simulink model "ee_solenoid_fem"  (R2022a)
settings: Solver=VariableStepAuto  StartTime=0.0  StopTime=0.1  FixedStep=2e-5  MaxStep=0.001  RelTol=1e-3  EnableMultiTasking=on
PreLoadFcn:
  | load ee_solenoid_fem_data
StopFcn:
  | ee_addSimlogTimeStamp(bdroot)
values from neighbouring files (symbols this model uses):
  lambda = 20    [ee_solenoid_fem_params.m]
  mass = 0.1    [ee_solenoid_fem_params.m]
  R = 14    [ee_solenoid_fem_params.m]
libraries: fl_lib x27, fl_ps_legacy_lib x10, nesl_utility x7, ee_lib x1
CloseFcn:
  | try,close(h1_ee_solenoid_fem),end
  | clear h1_ee_solenoid_fem
  | try,close(h2_ee_solenoid_fem),end
  | clear h2_ee_solenoid_fem
  | try,close(h3_ee_solenoid_fem),end
  | clear h3_ee_solenoid_fem
  | try,close(h4_ee_solenoid_fem),end
  | clear h4_ee_solenoid_fem
  | try,close(h5_ee_solenoid_fem),end
  | clear h5_ee_solenoid_fem
  | 
  | clear simlog_ee_solenoid_fem
  | clear logsout_ee_solenoid_fem
  | clear Coeff L R X a b current dLdx data_coeff dflux_dx dflux_dx1 dflux_dx2 dfluxdi dfluxdx f_c flux_linkage flux_linkage2 flux_x force force2 force_x i lambda mass oo ord p tout x x0 xmax xmin zz
Description:
  | Solenoid Parameterized with FEM Data
settings Model: Creator=The MathWorks, Inc.  LastModifiedBy=whatastarrynight
settings SolverCC: AlgebraicLoopSolver=TrustRegion
settings DataIOCC: LimitDataPoints=on  MaxDataPoints=10000  SaveFormat=Array  ReturnWorkspaceOutputs=off  SignalLoggingName=logsout_ee_solenoid_fem
settings OptimizationCC: ExpressionDepthLimit=2147483647  InitFltsAndDblsToZero=on  LifeSpan=inf
settings DebuggingCC: SaveWithParameterizedLinksMsg=none  UnderspecifiedInitializationDetection=Classic  MergeDetectMultiDrivingBlocksExec=none  SignalResolutionControl=TryResolveAllWithWarning  SolverPrmCheckMsg=warning  FcnCallInpInsideContextMsg=warning  UnconnectedInputMsg=warning  UnconnectedOutputMsg=warning  UnconnectedLineMsg=warning  StateNameClashWarn=warning  SFUnexpectedBacktrackingDiag=warning  SFNoUnconditionalDefaultTransitionDiag=warning  SFExecutionAtInitializationDiag=none  SFMachineParentedDataDiag=warning  ArithmeticOperatorsInVariantConditions=warning
settings HardwareCC: ProdBitPerPointer=32  ProdBitPerSizeT=32  ProdBitPerPtrDiffT=32  ProdLargestAtomicFloat=None  ProdIntDivRoundTo=Undefined  ProdEndianess=Unspecified  ProdWordSize=32  ProdHWDeviceType=32-bit Generic
settings ModelReferenceCC: PropagateSignalLabelsOutOfModel=off
settings SFSimCC: SimUseLocalCustomCode=off  CustomCodeUndefinedFunction=UseInterfaceOnly
settings RTWCC: RTWUseLocalCustomCode=off  DLArmComputeVersion=19.05
settings CodeAppCC: StateflowObjectComments=on
settings GRTTargetCC: TargetFcnLib=ansi_tfl_tmw.mat  TargetLangStandard=C89/C90 (ANSI)  CombineOutputUpdateFcns=off  GRTInterface=on
settings ConfigComp: CovMetricSettings=dw  CovSaveCumulativeToWorkspaceVar=on  CovSaveSingleToWorkspaceVar=on  CovExternalEMLEnable=off  CovSFcnEnable=off
settings SimscapeCC: SimscapeLogType=all  SimscapeLogSimulationStatistics=on  SimscapeLogToSDI=on  SimscapeLogName=simlog_ee_solenoid_fem  SimscapeLogDataHistory=10000

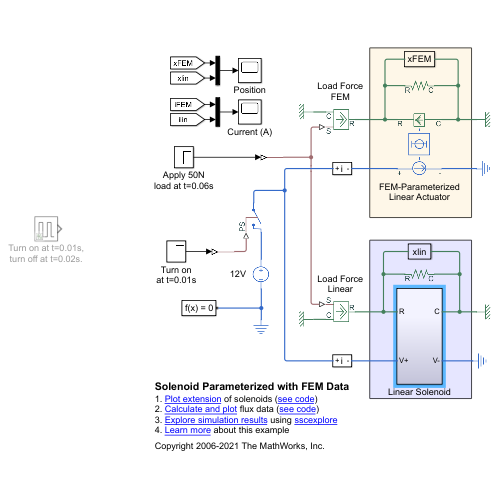
[thumbnail: Simulink's stored preview of the top-level diagram]
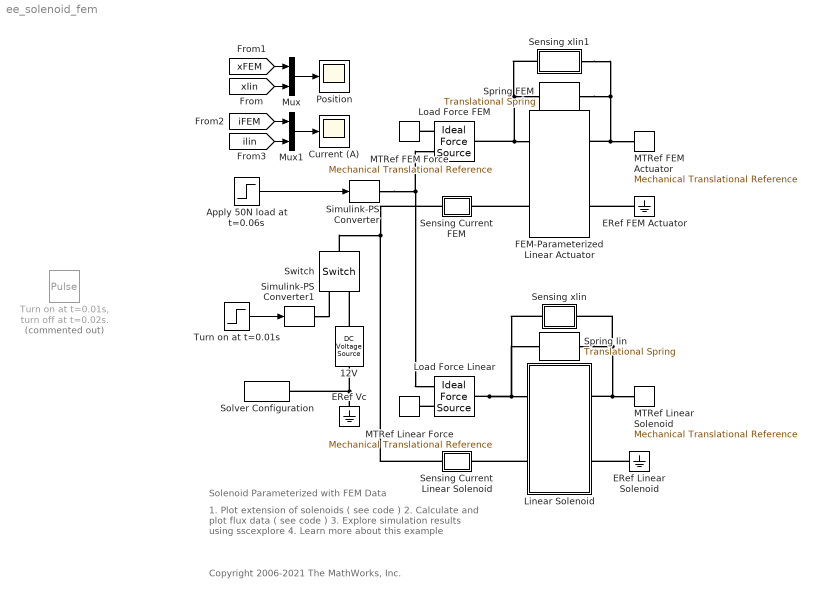
== system ee_solenoid_fem ==
  note: Solenoid Parameterized with FEM Data
  note: 1. Plot extension of solenoids ( see code )
      | 2. Calculate and plot flux data ( see code )
      | 3. Explore simulation results using sscexplore
      | 4. Learn more about this example
  note: Copyright 2006-2021 The MathWorks, Inc.
  12V : fl_lib/Electrical/Electrical Sources/DC Voltage Source  v0=12 V
      settings: SourceProductBaseCode=PW,SS,VE
  Apply 50N load at t=0.06s : Step  Time=0.06  After=50  SampleTime=0
  Current (A) : Scope
  ERef FEM Actuator : fl_lib/Electrical/Electrical Elements/Electrical Reference
      settings: SourceProductBaseCode=PW,SS,VE
  ERef Linear Solenoid : fl_lib/Electrical/Electrical Elements/Electrical Reference
      settings: SourceProductBaseCode=PW,SS,VE
  ERef Vc : fl_lib/Electrical/Electrical Elements/Electrical Reference
      settings: SourceProductBaseCode=PW,SS,VE
  FEM-Parameterized Linear Actuator : ee_lib/Electromechanical/Mechatronic Actuators/FEM-Parameterized Linear Actuator  src_type=2  iVec=current A  xVec=x m  dfluxdiMatrix=dfluxdi Wb/A  dfluxdxMatrix=dfluxdx Wb/m  FluxMatrix=flux_linkage Wb  calculate_force_matrix=ee.enum.enable.no  ForceMatrix=force N  cyclic=1  interp_method=1  extrap_method=1  R1=R Ohm  Rm=inf Ohm  lam=lambda N/(m/s)  Mass=mass kg  Xmin=xmin m  Xmax=xmax m  K_endstop=1e10 N/m  D_endstop=1e5 N/(m/s)  i_specify=off  i_priority=None  i=0 A  i_nominal_specify=off  i_nominal_unit=A  i_nominal_value=1  F_specify=off  F_priority=None  F=0 N  F_nominal_specify=off  F_nominal_unit=N  F_nominal_value=1  x_specify=on  x_priority=High  x=x0 m  x_nominal_specify=off  x_nominal_unit=mm  x_nominal_value=1  vel_specify=on  vel_priority=Low  vel=0 mm/s  vel_nominal_specify=off  vel_nominal_unit=mm/s  vel_nominal_value=1  magnetic_force_specify=off  magnetic_force_priority=None  magnetic_force=0 N  magnetic_force_nominal_specify=off  magnetic_force_nominal_unit=N  magnetic_force_nominal_value=1  alpha=3.93e-3 1/K  Tmeas=25 degC  thermal_mass=100 J/K  T_specify=off  T_priority=High  T=300 K  T_nominal_specify=off  T_nominal_unit=K  T_nominal_value=1
      settings: SourceProductBaseCode=PS  InternalSimscapePortConfiguration="{\"Bottom\":[],\"Left\":[{\"id\":\"p\",\"label\":\"+\",\"type\":\"foundation.electrical.electrical\"},{\"id\":\"R\",\"label\":\"R\",\"type\":\"foundation.mechanical.translational.translational\"}],\"Right\":[{\"id\":\"n\",\"label\":\"-\",\"type\":\"foundation.electrical.electrical\"},{\"id\":\"C\",\"label\":\"C\",\"type\":\"foundation.mechanical.translational.translational\"}],\"Top\":[]}"
  Linear Solenoid : Subsystem
  Load Force FEM : fl_lib/Mechanical/Mechanical Sources/Ideal Force Source
      settings: SourceProductBaseCode=PW,SS,VE
  Load Force Linear : fl_lib/Mechanical/Mechanical Sources/Ideal Force Source
      settings: SourceProductBaseCode=PW,SS,VE
  MTRef Linear Force : fl_lib/Mechanical/Translational Elements/Mechanical Translational Reference
      settings: SourceProductBaseCode=PW,SS,VE
  MTRef FEM Actuator : fl_lib/Mechanical/Translational Elements/Mechanical Translational Reference
      settings: SourceProductBaseCode=PW,SS,VE
  MTRef FEM Force : fl_lib/Mechanical/Translational Elements/Mechanical Translational Reference
      settings: SourceProductBaseCode=PW,SS,VE
  MTRef Linear Solenoid : fl_lib/Mechanical/Translational Elements/Mechanical Translational Reference
      settings: SourceProductBaseCode=PW,SS,VE
  Mux : Mux  Inputs=2
  Mux1 : Mux  Inputs=2
  Position : Scope
  Sensing Current FEM : Subsystem
      mask Display: disp('i')
  Sensing Current Linear Solenoid : Subsystem
      mask Display: disp('i')
  Sensing xlin : Subsystem
      mask Display: disp('xlin')
  Sensing xlin1 : Subsystem
      mask Display: disp('xFEM')
  Simulink-PS Converter : nesl_utility/Simulink-PS Converter  PhysicalDomain=network_engine_domain  SubClassName=ps_input  LeftPortType=input  RightPortType=output  PseudoPeriodic=off  Frequencies=[]  NoiseDistribution=none  NoiseParameters=[]  Unit=1  AffineConversion=off  FilteringAndDerivatives=zero  SimscapeFilterOrder=1  InputFilterTimeConstant=.001  UdotUserProvided=0
      settings: SourceProductBaseCode=SS,PW,VE
  Simulink-PS Converter1 : nesl_utility/Simulink-PS Converter  PhysicalDomain=network_engine_domain  SubClassName=ps_input  LeftPortType=input  RightPortType=output  PseudoPeriodic=off  Frequencies=[]  NoiseDistribution=none  NoiseParameters=[]  Unit=1  AffineConversion=off  FilteringAndDerivatives=zero  SimscapeFilterOrder=1  InputFilterTimeConstant=.001  UdotUserProvided=0
      settings: SourceProductBaseCode=SS,PW,VE
  Solver Configuration : nesl_utility/Solver Configuration  PhysicalDomain=network_engine_domain  SubClassName=solver  LeftPortType=input  RightPortType=generic  Tones=[]  Harmonics=[]  SimulateNoise=off  Profile=off  UseLocalSampling=off  EnableSwitchedLinearOptims=on  FrequencyDomain=off  UseCCode=off  RelTol=0.001  AbsTol=1e-06  MinStep=1e-09  ToWorkspace=off  RevertToSquareIcSolve=off  NumHomotopyIterations=100  PhasorMode=off  PhasorModeNumHarmonics=1  IndexReductionMethod=DerivativeReplacement  DoDC=off  ResidualTolerance=1e-9  UseLocalSolver=off  LocalSolverChoice=NE_TRAPEZOIDAL_ADVANCER  LocalSolverSampleTime=2e-5  DoFixedCost=off  MaxNonlinIter=12  MaxModeIter=2  ComputeImpulses=off  ImpulseIterations=2  LinearAlgebra=auto  LinearAlgebraNumThread=0  EquationFormulation=NE_TIME_EF  DelaysMemoryBudget=1024  AutomaticFiltering=on  FilteringTimeConstant=0.001  PartitionStorageMethod=AS_NEEDED  PartitionMemoryBudget=1024  PartitionMethod=FAST
      settings: SourceProductBaseCode=SS,PW,VE
  Spring FEM : fl_lib/Mechanical/Translational Elements/Translational Spring  spr_rate=200 N/m  v_specify=off  v_priority=High  v=0 m/s  v_nominal_specify=off  v_nominal_unit=m/s  v_nominal_value=1  f_specify=off  f_priority=High  f=0 N  f_nominal_specify=off  f_nominal_unit=N  f_nominal_value=1  x_specify=on  x_priority=High  x=0 mm  x_nominal_specify=off  x_nominal_unit=m  x_nominal_value=1
      settings: SourceProductBaseCode=PW,SS,VE
  Spring lin : fl_lib/Mechanical/Translational Elements/Translational Spring  spr_rate=200 N/m  v_specify=off  v_priority=High  v=0 m/s  v_nominal_specify=off  v_nominal_unit=m/s  v_nominal_value=1  f_specify=off  f_priority=High  f=0 N  f_nominal_specify=off  f_nominal_unit=N  f_nominal_value=1  x_specify=on  x_priority=High  x=0 mm  x_nominal_specify=off  x_nominal_unit=m  x_nominal_value=1
      settings: SourceProductBaseCode=PW,SS,VE
  Switch : fl_lib/Electrical/Electrical Elements/Switch  R_closed=0.01 Ohm  G_open=1e-8 1/Ohm  Threshold=0  i_specify=off  i_priority=High  i=0 A  i_nominal_specify=off  i_nominal_unit=A  i_nominal_value=1  v_specify=off  v_priority=High  v=0 V  v_nominal_specify=off  v_nominal_unit=V  v_nominal_value=1
      settings: SourceProductBaseCode=PW,SS,VE
  Turn on at t=0.01s : Step  Time=0.01  SampleTime=0
  "Turn on at t=0.01s, turn off at t=0.02s." : DiscretePulseGenerator  Commented=on  PulseType=Time based  Period=0.1  PulseWidth=10  PhaseDelay=0.01
  wires:
  Apply 50N load at t=0.06s/1 -> Simulink-PS Converter/1
  Mux/1 -> Position/1
  Mux1/1 -> Current (A)/1
  [xlin] -> Mux/2
  [xFEM] -> Mux/1
  [iFEM] -> Mux1/1
  [ilin] -> Mux1/2
  Turn on at t=0.01s/1 -> Simulink-PS Converter1/1
  connections:
  Linear Solenoid/LConn2 -- Sensing Current Linear Solenoid/RConn1
  Simulink-PS Converter1/RConn1 -- Switch/RConn1
  12V/LConn1 -- Switch/RConn2
  ERef Vc/LConn1 -- 12V/RConn1 -- Solver Configuration/RConn1
  ERef FEM Actuator/LConn1 -- FEM-Parameterized Linear Actuator/RConn1
  FEM-Parameterized Linear Actuator/LConn2 -- Load Force FEM/LConn1 -- Sensing xlin1/LConn1 -- Spring FEM/LConn1
  Spring FEM/RConn1 -- Sensing xlin1/RConn1 -- MTRef FEM Actuator/LConn1 -- FEM-Parameterized Linear Actuator/RConn2
  Load Force FEM/RConn2 -- MTRef FEM Force/LConn1
  Load Force Linear/RConn2 -- MTRef Linear Force/LConn1
  Simulink-PS Converter/RConn1 -- Load Force FEM/RConn1 -- Load Force Linear/RConn1
  Spring lin/RConn1 -- Sensing xlin/RConn1 -- MTRef Linear Solenoid/LConn1 -- Linear Solenoid/RConn1
  ERef Linear Solenoid/LConn1 -- Linear Solenoid/RConn2
  Load Force Linear/LConn1 -- Sensing xlin/LConn1 -- Spring lin/LConn1 -- Linear Solenoid/LConn1
  FEM-Parameterized Linear Actuator/LConn1 -- Sensing Current FEM/RConn1
  Sensing Current FEM/LConn1 -- Sensing Current Linear Solenoid/LConn1 -- Switch/LConn1

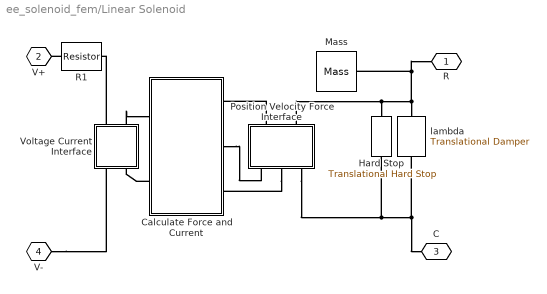
== system ee_solenoid_fem/Linear Solenoid ==
  Calculate Force and Current : Subsystem
  Hard Stop : fl_lib/Mechanical/Translational Elements/Translational Hard Stop  upper_bnd=xmax m  lower_bnd=xmin m  stiff_up=1e+10 N/m  stiff_low=1e+10 N/m  D_up=1e5 N/(m/s)  D_low=1e5 N/(m/s)  model=3  transition=0.1 mm  v_specify=off  v_priority=High  v=0 m/s  v_nominal_specify=off  v_nominal_unit=m/s  v_nominal_value=1  f_specify=off  f_priority=High  f=0 N  f_nominal_specify=off  f_nominal_unit=N  f_nominal_value=1  x_specify=on  x_priority=High  x=x0 m  x_nominal_specify=off  x_nominal_unit=m  x_nominal_value=1
      settings: SourceProductBaseCode=PW,SS,VE
  Mass : fl_lib/Mechanical/Translational Elements/Mass  mass=mass kg  num_ports=foundation.enum.numPorts2.one  v_specify=on  v_priority=High  v=0 m/s  v_nominal_specify=off  v_nominal_unit=m/s  v_nominal_value=1  f_specify=off  f_priority=High  f=0 N  f_nominal_specify=off  f_nominal_unit=N  f_nominal_value=1
      settings: SourceProductBaseCode=PW,SS,VE
  Position Velocity Force Interface : Subsystem
  R1 : fl_lib/Electrical/Electrical Elements/Resistor  R=R Ohm  i_specify=off  i_priority=High  i=0 A  i_nominal_specify=off  i_nominal_unit=A  i_nominal_value=1  v_specify=off  v_priority=High  v=0 V  v_nominal_specify=off  v_nominal_unit=V  v_nominal_value=1
      settings: SourceProductBaseCode=PW,SS,VE
  Voltage Current Interface : Subsystem
  lambda : fl_lib/Mechanical/Translational Elements/Translational Damper  D=lambda N/(m/s)  v_specify=off  v_priority=High  v=0 m/s  v_nominal_specify=off  v_nominal_unit=m/s  v_nominal_value=1  f_specify=off  f_priority=High  f=0 N  f_nominal_specify=off  f_nominal_unit=N  f_nominal_value=1
      settings: SourceProductBaseCode=PW,SS,VE
  R : PMIOPort  Side=Left
  V+ : PMIOPort  Port=2  Side=Left
  C : PMIOPort  Port=3  Side=Right
  V- : PMIOPort  Port=4  Side=Right
  connections:
  Hard Stop/RConn1 -- lambda/RConn1 -- C/RConn1 -- Position Velocity Force Interface/RConn3
  R1/LConn1 -- V+/RConn1
  lambda/LConn1 -- R/RConn1 -- Mass/LConn1 -- Position Velocity Force Interface/LConn2 -- Hard Stop/LConn1
  Position Velocity Force Interface/LConn1 -- Calculate Force and Current/RConn1
  Calculate Force and Current/RConn2 -- Position Velocity Force Interface/RConn1
  Position Velocity Force Interface/RConn2 -- Calculate Force and Current/RConn3
  Voltage Current Interface/LConn1 -- R1/RConn1
  V-/RConn1 -- Voltage Current Interface/RConn1
  Voltage Current Interface/LConn2 -- Calculate Force and Current/LConn1
  Calculate Force and Current/LConn2 -- Voltage Current Interface/RConn2

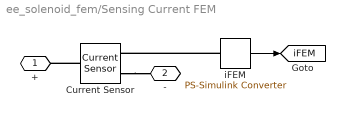
== system ee_solenoid_fem/Sensing Current FEM ==
  Current Sensor : fl_lib/Electrical/Electrical Sensors/Current Sensor
      settings: SourceProductBaseCode=PW,SS,VE
  iFEM : nesl_utility/PS-Simulink Converter  PhysicalDomain=network_engine_domain  SubClassName=ps_output  LeftPortType=input  RightPortType=output  PseudoPeriodic=off  Frequencies=[]  VectorFormat=1-D array  Unit=1  AffineConversion=off
      settings: SourceProductBaseCode=SS,PW,VE
  + : PMIOPort  Side=Left
  - : PMIOPort  Port=2  Side=Right
  tag scope: iFEM=global
  wires:
  iFEM/1 -> [iFEM]
  connections:
  iFEM/LConn1 -- Current Sensor/RConn1
  Current Sensor/LConn1 -- +/RConn1
  Current Sensor/RConn2 -- -/RConn1

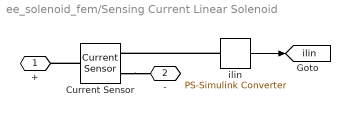
== system ee_solenoid_fem/Sensing Current Linear Solenoid ==
  Current Sensor : fl_lib/Electrical/Electrical Sensors/Current Sensor
      settings: SourceProductBaseCode=PW,SS,VE
  ilin : nesl_utility/PS-Simulink Converter  PhysicalDomain=network_engine_domain  SubClassName=ps_output  LeftPortType=input  RightPortType=output  PseudoPeriodic=off  Frequencies=[]  VectorFormat=1-D array  Unit=1  AffineConversion=off
      settings: SourceProductBaseCode=SS,PW,VE
  + : PMIOPort  Side=Left
  - : PMIOPort  Port=2  Side=Right
  tag scope: ilin=global
  wires:
  ilin/1 -> [ilin]
  connections:
  Current Sensor/RConn2 -- -/RConn1
  Current Sensor/LConn1 -- +/RConn1
  ilin/LConn1 -- Current Sensor/RConn1

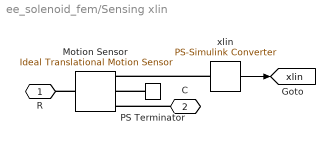
== system ee_solenoid_fem/Sensing xlin ==
  Motion Sensor : fl_lib/Mechanical/Mechanical Sensors/Ideal Translational Motion Sensor  offset=x0 m
      settings: SourceProductBaseCode=PW,SS,VE
  PS Terminator : fl_lib/Physical Signals/Sinks/PS Terminator
      settings: SourceProductBaseCode=PW,SS,VE
  xlin : nesl_utility/PS-Simulink Converter  PhysicalDomain=network_engine_domain  SubClassName=ps_output  LeftPortType=input  RightPortType=output  PseudoPeriodic=off  Frequencies=[]  VectorFormat=1-D array  Unit=mm  AffineConversion=off
      settings: SourceProductBaseCode=SS,PW,VE
  R : PMIOPort  Side=Left
  C : PMIOPort  Port=2  Side=Right
  tag scope: xlin=global
  wires:
  xlin/1 -> [xlin]
  connections:
  C/RConn1 -- Motion Sensor/RConn1
  PS Terminator/LConn1 -- Motion Sensor/RConn2
  Motion Sensor/LConn1 -- R/RConn1
  xlin/LConn1 -- Motion Sensor/RConn3

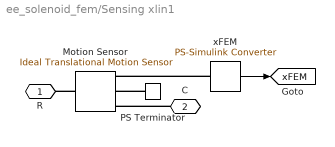
== system ee_solenoid_fem/Sensing xlin1 ==
  Motion Sensor : fl_lib/Mechanical/Mechanical Sensors/Ideal Translational Motion Sensor  offset=x0 m
      settings: SourceProductBaseCode=PW,SS,VE
  PS Terminator : fl_lib/Physical Signals/Sinks/PS Terminator
      settings: SourceProductBaseCode=PW,SS,VE
  xFEM : nesl_utility/PS-Simulink Converter  PhysicalDomain=network_engine_domain  SubClassName=ps_output  LeftPortType=input  RightPortType=output  PseudoPeriodic=off  Frequencies=[]  VectorFormat=1-D array  Unit=mm  AffineConversion=off
      settings: SourceProductBaseCode=SS,PW,VE
  R : PMIOPort  Side=Left
  C : PMIOPort  Port=2  Side=Right
  tag scope: xFEM=global
  wires:
  xFEM/1 -> [xFEM]
  connections:
  xFEM/LConn1 -- Motion Sensor/RConn3
  Motion Sensor/LConn1 -- R/RConn1
  PS Terminator/LConn1 -- Motion Sensor/RConn2
  C/RConn1 -- Motion Sensor/RConn1

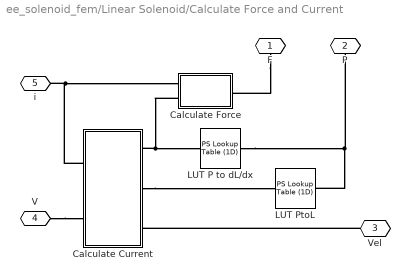
== system ee_solenoid_fem/Linear Solenoid/Calculate Force and Current ==
  Calculate Current : Subsystem
  Calculate Force : Subsystem
  LUT P to dL/dx : fl_ps_legacy_lib/Legacy Physical Signals/Lookup Tables/PS Lookup Table (1D)  x=x  f=dLdx  interp_method=1  extrap_method=1
      settings: SourceProductBaseCode=PW,SS,VE  InternalSimscapePortConfiguration="{\"Bottom\":[],\"Left\":[{\"id\":\"I\",\"label\":\"x\",\"type\":\"input\"}],\"Right\":[{\"id\":\"O\",\"label\":\"f\",\"type\":\"output\"}],\"Top\":[]}"
  LUT PtoL : fl_ps_legacy_lib/Legacy Physical Signals/Lookup Tables/PS Lookup Table (1D)  x=x  f=L  interp_method=1  extrap_method=1
      settings: SourceProductBaseCode=PW,SS,VE  InternalSimscapePortConfiguration="{\"Bottom\":[],\"Left\":[{\"id\":\"I\",\"label\":\"x\",\"type\":\"input\"}],\"Right\":[{\"id\":\"O\",\"label\":\"f\",\"type\":\"output\"}],\"Top\":[]}"
  F : PMIOPort  Side=Right
  P : PMIOPort  Port=2  Side=Right
  Vel : PMIOPort  Port=3  Side=Right
  V : PMIOPort  Port=4  Side=Left
  i : PMIOPort  Port=5  Side=Left
  connections:
  LUT P to dL/dx/LConn1 -- LUT PtoL/LConn1 -- P/RConn1
  F/RConn1 -- Calculate Force/RConn1
  Vel/RConn1 -- Calculate Current/LConn3
  Calculate Force/LConn2 -- LUT P to dL/dx/RConn1 -- Calculate Current/LConn1
  Calculate Current/LConn2 -- LUT PtoL/RConn1
  V/RConn1 -- Calculate Current/RConn2
  Calculate Current/RConn1 -- Calculate Force/LConn1 -- i/RConn1

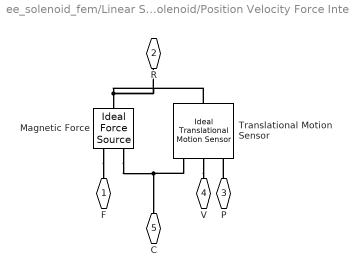
== system ee_solenoid_fem/Linear Solenoid/Position Velocity Force Interface ==
  Magnetic Force : fl_lib/Mechanical/Mechanical Sources/Ideal Force Source
      settings: SourceProductBaseCode=PW,SS,VE
  Translational Motion Sensor : fl_lib/Mechanical/Mechanical Sensors/Ideal Translational Motion Sensor  offset=x0 m
      settings: SourceProductBaseCode=PW,SS,VE
  F : PMIOPort  Side=Left
  R : PMIOPort  Port=2  Side=Left
  P : PMIOPort  Port=3  Side=Right
  V : PMIOPort  Port=4  Side=Right
  C : PMIOPort  Port=5  Side=Right
  connections:
  Translational Motion Sensor/RConn1 -- Magnetic Force/RConn2 -- C/RConn1
  P/RConn1 -- Translational Motion Sensor/RConn3
  Magnetic Force/LConn1 -- Translational Motion Sensor/LConn1 -- R/RConn1
  Translational Motion Sensor/RConn2 -- V/RConn1
  Magnetic Force/RConn1 -- F/RConn1

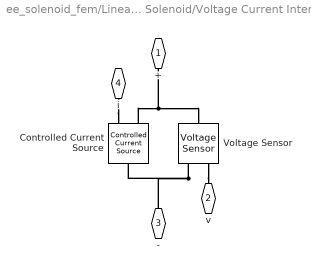
== system ee_solenoid_fem/Linear Solenoid/Voltage Current Interface ==
  Controlled Current Source : fl_lib/Electrical/Electrical Sources/Controlled Current Source
      settings: SourceProductBaseCode=PW,SS,VE
  Voltage Sensor : fl_lib/Electrical/Electrical Sensors/Voltage Sensor
      settings: SourceProductBaseCode=PW,SS,VE
  + : PMIOPort  Side=Left
  v : PMIOPort  Port=2  Side=Left
  - : PMIOPort  Port=3  Side=Right
  i : PMIOPort  Port=4  Side=Right
  connections:
  i/RConn1 -- Controlled Current Source/RConn1
  Voltage Sensor/RConn1 -- v/RConn1
  Voltage Sensor/RConn2 -- Controlled Current Source/LConn1 -- -/RConn1
  Controlled Current Source/RConn2 -- +/RConn1 -- Voltage Sensor/LConn1

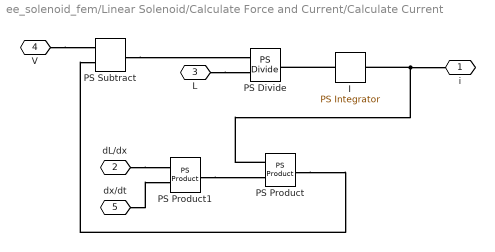
== system ee_solenoid_fem/Linear Solenoid/Calculate Force and Current/Calculate Current ==
  I : fl_ps_legacy_lib/Legacy Physical Signals/Linear Operators/PS Integrator  x0=0
      settings: SourceProductBaseCode=PW,SS,VE  InternalSimscapePortConfiguration="{\"Bottom\":[],\"Left\":[{\"id\":\"I\",\"label\":\"\",\"type\":\"input\"}],\"Right\":[{\"id\":\"O\",\"label\":\"\",\"type\":\"output\"}],\"Top\":[]}"
  PS Divide : fl_ps_legacy_lib/Legacy Physical Signals/Functions/PS Divide
      settings: SourceProductBaseCode=PW,SS,VE  InternalSimscapePortConfiguration="{\"Bottom\":[],\"Left\":[{\"id\":\"I1\",\"label\":\"\",\"type\":\"input\"},{\"id\":\"I2\",\"label\":\"\",\"type\":\"input\"}],\"Right\":[{\"id\":\"O\",\"label\":\"\",\"type\":\"output\"}],\"Top\":[]}"
  PS Product : fl_ps_legacy_lib/Legacy Physical Signals/Functions/PS Product
      settings: SourceProductBaseCode=PW,SS,VE
  PS Product1 : fl_ps_legacy_lib/Legacy Physical Signals/Functions/PS Product
      settings: SourceProductBaseCode=PW,SS,VE
  PS Subtract : fl_ps_legacy_lib/Legacy Physical Signals/Functions/PS Subtract
      settings: SourceProductBaseCode=PW,SS,VE
  i : PMIOPort  Side=Right
  dL/dx : PMIOPort  Port=2  Side=Left
  L : PMIOPort  Port=3  Side=Left
  V : PMIOPort  Port=4  Side=Right
  dx/dt : PMIOPort  Port=5  Side=Left
  connections:
  I/LConn1 -- PS Divide/RConn1
  PS Subtract/RConn1 -- PS Divide/LConn1
  PS Product1/RConn1 -- PS Product/LConn2
  PS Product/RConn1 -- PS Subtract/LConn2
  L/RConn1 -- PS Divide/LConn2
  V/RConn1 -- PS Subtract/LConn1
  dL/dx/RConn1 -- PS Product1/LConn1
  dx/dt/RConn1 -- PS Product1/LConn2
  PS Product/LConn1 -- i/RConn1 -- I/RConn1

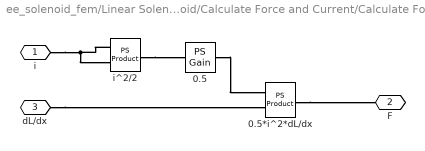
== system ee_solenoid_fem/Linear Solenoid/Calculate Force and Current/Calculate Force ==
  0.5 : fl_ps_legacy_lib/Legacy Physical Signals/Functions/PS Gain  gain=0.5
      settings: SourceProductBaseCode=PW,SS,VE
  0.5*i^2*dL/dx : fl_ps_legacy_lib/Legacy Physical Signals/Functions/PS Product
      settings: SourceProductBaseCode=PW,SS,VE
  i^2/2 : fl_ps_legacy_lib/Legacy Physical Signals/Functions/PS Product
      settings: SourceProductBaseCode=PW,SS,VE
  i : PMIOPort  Side=Left
  F : PMIOPort  Port=2  Side=Right
  dL/dx : PMIOPort  Port=3  Side=Left
  connections:
  i^2/2/LConn1 -- i^2/2/LConn2 -- i/RConn1
  0.5*i^2*dL/dx/RConn1 -- F/RConn1
  dL/dx/RConn1 -- 0.5*i^2*dL/dx/LConn2
  i^2/2/RConn1 -- 0.5/LConn1
  0.5/RConn1 -- 0.5*i^2*dL/dx/LConn1
